simulink library "calcPathLengthOverRange"  (R2022a)
settings: Solver=VariableStepAuto  StartTime=0.0  StopTime=10.0  RelTol=1e-3
settings Model: Creator=Ayaz  LastModifiedBy=lhill8
settings SolverCC: AlgebraicLoopSolver=TrustRegion
settings DebuggingCC: UnconnectedInputMsg=warning  UnconnectedOutputMsg=warning  UnconnectedLineMsg=warning  SFMachineParentedDataDiag=warning

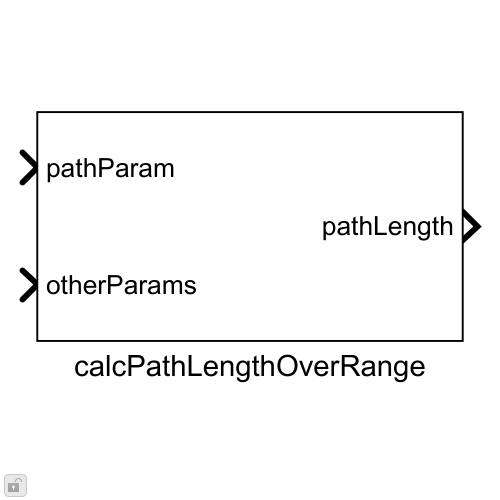
[thumbnail: Simulink's stored preview of the top-level diagram]
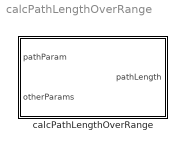
== system calcPathLengthOverRange ==
  calcPathLengthOverRange : Subsystem

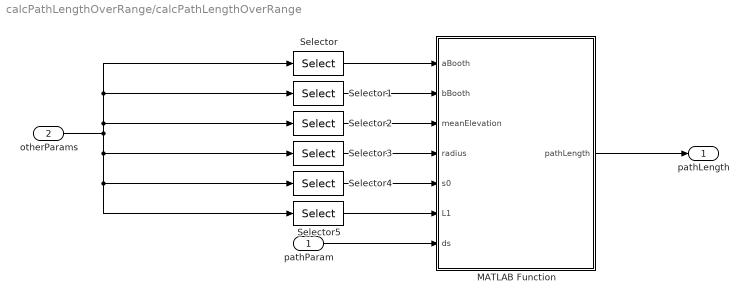
== system calcPathLengthOverRange/calcPathLengthOverRange ==
  pathParam : Inport
  otherParams : Inport  Port=2
  MATLAB Function : MATLAB Function  TreatAsAtomicUnit=on
  Selector : Selector  InputPortWidth=6  IndexOptions=Index vector (dialog)  Indices=1  OutputSizes=1
  Selector1 : Selector  InputPortWidth=6  IndexOptions=Index vector (dialog)  Indices=2  OutputSizes=1
  Selector2 : Selector  InputPortWidth=6  IndexOptions=Index vector (dialog)  Indices=3  OutputSizes=1
  Selector3 : Selector  InputPortWidth=6  IndexOptions=Index vector (dialog)  Indices=4  OutputSizes=1
  Selector4 : Selector  InputPortWidth=6  IndexOptions=Index vector (dialog)  Indices=5  OutputSizes=1
  Selector5 : Selector  InputPortWidth=6  IndexOptions=Index vector (dialog)  Indices=6  OutputSizes=1
  pathLength : Outport
  wires:
  MATLAB Function/1(pathLength) -> pathLength/1
  otherParams/1 -> Selector3/1, Selector4/1, Selector5/1, Selector2/1, Selector1/1, Selector/1
  Selector5/1 -> MATLAB Function/6(L1)
  Selector4/1 -> MATLAB Function/5(s0)
  Selector3/1 -> MATLAB Function/4(radius)
  Selector2/1 -> MATLAB Function/3(meanElevation)
  Selector1/1 -> MATLAB Function/2(bBooth)
  Selector/1 -> MATLAB Function/1(aBooth)
  pathParam/1 -> MATLAB Function/7(ds)

== matlab function calcPathLengthOverRange/MATLAB Function ==
  data: aBooth input; pathLength output; bBooth input; meanElevation input; radius input; s0 input; L1 input; ds input
function pathLength = calcTargetDistance(aBooth,bBooth,meanElevation,radius,s0,L1,ds)

pathLength = calcTargetDistance(aBooth,bBooth,meanElevation,radius,s0,L1,ds);

end
